simulink model "PKE_expr"  (R2015b)
settings: Solver=ode45  StartTime=0.0  StopTime=1000  RelTol=1e-3
values from neighbouring files (symbols this model uses):
  B = sum(bet)    [PKE_general.m]    (also in Parameters_MSBR_new_nodal.m = 0.532280235372; Parameters_steady_state.m = 0.266140117686; pke_driver.m)
  bet = [0.000229,0.000832,0.000710,0.000852,0.000171,0.000102]'    [PKE_general.m]    (also in pke_driver.m = [2.290E-04, 8.320E-04, 7.100E-04, 8.520E-04, 1.710E-04, 1.02)
  L = 0.0005    [PKE_general.m]    (also in pke_driver.m = 0.00033)
  lam = [0.0126,0.0337,0.139,0.325,1.13,2.50]'    [PKE_general.m]    (also in Parameters_Core_PHE.m = [1.260E-02, 3.370E-02, 1.390E-01, 3.250E-01, 1.130E+00, 2.50; Parameters_Core_PHE_FEHE.m = [1.260E-02, 3.370E-02, 1.390E-01, 3.250E-01, 1.130E+00, 2.50; Parameters_MSBR.m = [1.260E-02, 3.370E-02, 1.390E-01, 3.250E-01, 1.130E+00, 2.50; Parameters_MSBR_Brayton.m = [1.260E-02, 3.370E-02, 1.390E-01, 3.250E-01, 1.130E+00, 2.50)
  y0 = [nt,Ct(1),Ct(2),Ct(3),Ct(4),Ct(5),Ct(6)]'    [PKE_general.m]    (also in pke_driver.m = [nt_0;Ct_0])
settings Model: Creator=VIKRAM SINGH  LastModifiedBy=mlish
settings DataIOCC: LimitDataPoints=off  SaveFormat=Array
settings DebuggingCC: SolverPrmCheckMsg=warning
settings HardwareCC: ProdBitPerPointer=32  ProdLargestAtomicFloat=None  ProdIntDivRoundTo=Undefined  ProdEndianess=Unspecified  ProdWordSize=32  ProdHWDeviceType=32-bit Generic
settings GRTTargetCC: GeneratePreprocessorConditionals=Disable all
settings ConfigComp: CovModelRefEnable=Off  CovSFcnEnable=off

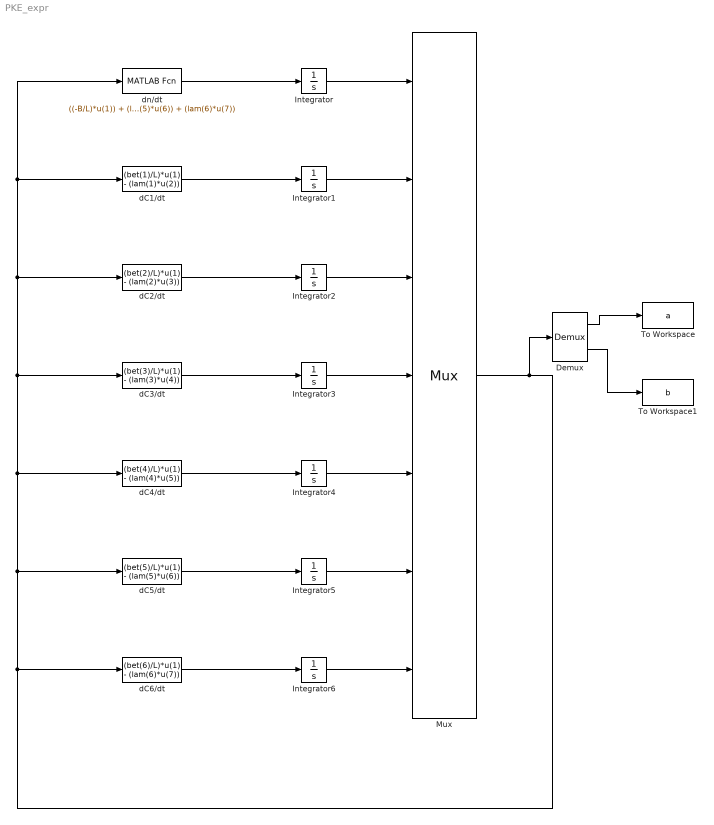
== system PKE_expr ==
  Demux : Demux  Outputs=[1,6]
  Integrator : Integrator  InitialCondition=y0(1)
  Integrator1 : Integrator  InitialCondition=y0(2)
  Integrator2 : Integrator  InitialCondition=y0(3)
  Integrator3 : Integrator  InitialCondition=y0(4)
  Integrator4 : Integrator  InitialCondition=y0(5)
  Integrator5 : Integrator  InitialCondition=y0(6)
  Integrator6 : Integrator  InitialCondition=y0(7)
  Mux : Mux  Inputs=7
      settings: DisplayOption=signals
  To Workspace : ToWorkspace  VariableName=a  SampleTime=-1
  To Workspace1 : ToWorkspace  VariableName=b  SampleTime=-1
  dC1/dt : MATLABFcn  MATLABFcn=(bet(1)/L)*u(1) - (lam(1)*u(2))
  dC2/dt : MATLABFcn  MATLABFcn=(bet(2)/L)*u(1) - (lam(2)*u(3))
  dC3/dt : MATLABFcn  MATLABFcn=(bet(3)/L)*u(1) - (lam(3)*u(4))
  dC4/dt : MATLABFcn  MATLABFcn=(bet(4)/L)*u(1) - (lam(4)*u(5))
  dC5/dt : MATLABFcn  MATLABFcn=(bet(5)/L)*u(1) - (lam(5)*u(6))
  dC6/dt : MATLABFcn  MATLABFcn=(bet(6)/L)*u(1) - (lam(6)*u(7))
  dn/dt : MATLABFcn  MATLABFcn=((-B/L)*u(1)) + (lam(1)*u(2)) + (lam(2)*u(3)) + (lam(3)*u(4)) + (lam(4)*u(5)) + (lam(5)*u(6)) + (lam(6)*u(7))
  wires:
  dn/dt/1 -> Integrator/1
  dC1/dt/1 -> Integrator1/1
  dC2/dt/1 -> Integrator2/1
  dC3/dt/1 -> Integrator3/1
  dC4/dt/1 -> Integrator4/1
  dC5/dt/1 -> Integrator5/1
  dC6/dt/1 -> Integrator6/1
  Mux/1 -> Demux/1, dC5/dt/1, dC4/dt/1, dC2/dt/1, dC1/dt/1, dn/dt/1, dC3/dt/1, dC6/dt/1
  Integrator/1 -> Mux/1
  Integrator1/1 -> Mux/2
  Integrator2/1 -> Mux/3
  Integrator3/1 -> Mux/4
  Integrator4/1 -> Mux/5
  Integrator5/1 -> Mux/6
  Integrator6/1 -> Mux/7
  Demux/1 -> To Workspace/1
  Demux/2 -> To Workspace1/1
